simulink model "Fig511"  (R2014b)
settings: Solver=ode3  StartTime=0.0  StopTime=.262144  FixedStep=1e-6  RelTol=1e-3
libraries: commseqgen2 x1
settings Model: Creator=Silage  LastModifiedBy=Silage

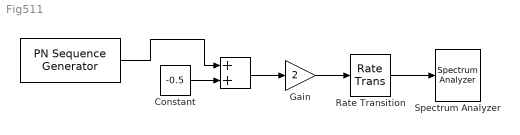
== system Fig511 ==
  " " : commseqgen2/PN Sequence Generator  poly=[1 0 0 1 1]  ini_sta=[1 0 0 1]  outBitMaskSource=Dialog parameter  shift=0  outVarSiz=off  maxOutSizeMode=Dialog parameter  maxOutSize=[10 1]  Ts=1e-3  frameBased=off  sampPerFrame=1  reset=off  bitPackedOutputs=off  outDataType=double  numPackedBits=8  bitPackDataSigned=off  bitPackedOutDType=double
  "    " : Sum
  Constant : Constant  Value=-0.5
  Gain : Gain  Gain=2
  Rate Transition : RateTransition  OutPortSampleTime=1e-6
  Spectrum Analyzer : SpectrumAnalyzer
  wires:
  " "/1 -> "    "/1
  Constant/1 -> "    "/2
  "    "/1 -> Gain/1
  Gain/1 -> Rate Transition/1
  Rate Transition/1 -> Spectrum Analyzer/1
